simulink model "Part4_SlidingMode"  (R2018a)
settings: Solver=ode45  StartTime=0.0  StopTime=2  RelTol=1e-3
values from neighbouring files (symbols this model uses):
  qqs = [t' qq]    [trajCircle.m]    (also in trajLine.m)
libraries: simulink x1, dspmathops x1, roblocks x1
settings Model: Creator=Francesco  LastModifiedBy=Francesco

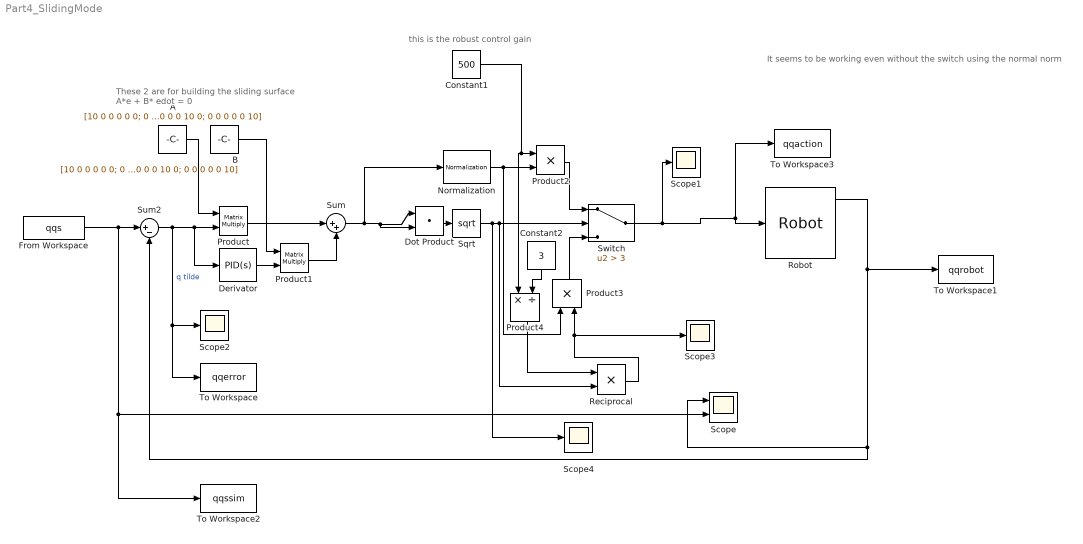
== system Part4_SlidingMode ==
  note: this is the robust control gain
  note: These 2 are for building the sliding surface
      | A*e + B* edot = 0
  note: It seems to be working even without the switch using the normal norm
  A : Constant  Value=[10 0 0 0 0 0; 0 10 0 0 0 0; 0 0 10 0 0 0; 0 0 0 10 0 0; 0 0 0 0 10 0; 0 0 0 0 0 10]
  B : Constant  Value=[10 0 0 0 0 0; 0 10 0 0 0 0; 0 0 10 0 0 0; 0 0 0 10 0 0; 0 0 0 0 10 0; 0 0 0 0 0 10]
  Constant1 : Constant  Value=500
  Constant2 : Constant  Value=3
  "Derivator " : simulink/Continuous/PID Controller  Controller=PID  TimeDomain=Continuous-time  SampleTime=-1  IntegratorMethod=Forward Euler  FilterMethod=Forward Euler  Form=Parallel  UseFilter=on  ControllerParametersSource=internal  P=0  I=0  D=1  N=100  InitialConditionSource=internal  InitialConditionForIntegrator=0  InitialConditionForFilter=0  ExternalReset=none  LimitOutput=off  UpperSaturationLimit=inf  LowerSaturationLimit=-inf  LinearizeAsGain=on  AntiWindupMode=none  Kb=1  TrackingMode=off  Kt=1  PParamMin=[]  PParamMax=[]  IParamMin=[]  IParamMax=[]  DParamMin=[]  DParamMax=[]  NParamMin=[]  NParamMax=[]  KbParamMin=[]  KbParamMax=[]  KtParamMin=[]  KtParamMax=[]  POutMin=[]  POutMax=[]  IOutMin=[]  IOutMax=[]  DOutMin=[]  DOutMax=[]  NOutMin=[]  NOutMax=[]  KbOutMin=[]  KbOutMax=[]  KtOutMin=[]  KtOutMax=[]  IntegratorOutMin=[]  IntegratorOutMax=[]  FilterOutMin=[]  FilterOutMax=[]  SumOutMin=[]  SumOutMax=[]  SumI1OutMin=[]  SumI1OutMax=[]  SumI2OutMin=[]  SumI2OutMax=[]  SumI3OutMin=[]  SumI3OutMax=[]  SumDOutMin=[]  SumDOutMax=[]  SaturationOutMin=[]  SaturationOutMax=[]  IntegratorContinuousStateAttributes=''  IntegratorStateMustResolveToSignalObject=off  IntegratorRTWStateStorageClass=Auto  FilterContinuousStateAttributes=''  FilterStateMustResolveToSignalObject=off  FilterRTWStateStorageClass=Auto  DifferentiatorICPrevScaledInput=0  DifferentiatorOutMin=[]  DifferentiatorOutMax=[]  FilterDiffOutCoefMin=[]  FilterDiffOutCoefMax=[]  SumDenOutMin=[]  SumDenOutMax=[]  SumNumOutMin=[]  SumNumOutMax=[]  ReciprocalOutMin=[]  ReciprocalOutMax=[]  DivideOutMin=[]  DivideOutMax=[]  TunerSelectOption=Transfer Function Based (PID Tuner App)
  Dot Product : DotProduct  InputSameDT=on  OutDataTypeStr=Inherit: Inherit via internal rule
  From Workspace : FromWorkspace  VariableName=qqs  SampleTime=0
  Normalization : dspmathops/Normalization  NormType=2-norm  Bias=1e-10  NormOver=Each column  Dimension=1  roundingMode=Floor  overflowMode=off  accumDataTypeStr=Inherit: Same as product output  accumLastDataTypeStr=Inherit: Same as product output  outputDataTypeStr=Inherit: Same as product output  outputMin=[]  outputMax=[]  outputLastDataTypeStr=Inherit: Same as product output
      settings: SourceProductName=DSP System Toolbox
  Product : Product  Multiplication=Matrix(*)
  Product1 : Product  Multiplication=Matrix(*)
  Product2 : Product
  Product3 : Product
  Product4 : Product  Inputs=*/
  Reciprocal : Product
  Robot : roblocks/Arm/Robot  robot=p560Unc  q0=qqs(1, 2:7)
  Scope : Scope  NumInputPorts=2
  Scope{1..4} (4 alike) : Scope
  Sqrt : Sqrt  SaturateOnIntegerOverflow=on
  Sum : Sum  Inputs=|++
  Sum2 : Sum  Inputs=|+-
  Switch : Switch  Criteria=u2 > Threshold  Threshold=3
  To Workspace : ToWorkspace  VariableName=qqerror  SaveFormat=Structure With Time  SampleTime=-1
  To Workspace1 : ToWorkspace  VariableName=qqrobot  SaveFormat=Structure With Time  SampleTime=-1
  To Workspace2 : ToWorkspace  VariableName=qqssim  SaveFormat=Structure With Time  SampleTime=-1
  To Workspace3 : ToWorkspace  VariableName=qqaction  SaveFormat=Structure With Time  SampleTime=-1
  wires:
  Robot/1 -> Scope/1, Sum2/2, To Workspace1/1
  Product2/1 -> Switch/1
  Sum2/1 -> Scope2/1, To Workspace/1, "Derivator "/1, Product/2  "q tilde"
  Constant1/1 -> Product2/1, Product4/1
  "Derivator "/1 -> Product1/2
  Product/1 -> Sum/1
  Product1/1 -> Sum/2
  A/1 -> Product/1
  B/1 -> Product1/1
  Sqrt/1 -> Reciprocal/2, Switch/2, Scope4/1
  Switch/1 -> Scope1/1, To Workspace3/1, Robot/1
  From Workspace/1 -> To Workspace2/1, Scope/2, Sum2/1
  Constant2/1 -> Product4/2
  Product4/1 -> Reciprocal/1
  Reciprocal/1 -> Scope3/1, Product3/2
  Dot Product/1 -> Sqrt/1
  Sum/1 -> Normalization/1, Dot Product/1, Dot Product/2
  Product3/1 -> Switch/3
  Normalization/1 -> Product3/1, Product2/2
